simulink model "Cessna_6DOF_Wind_trim"  (Simulink 8.6)
settings: Solver=ode45  StartTime=0.0  StopTime=10.0  RelTol=1e-3
values from neighbouring files (symbols this model uses):
  alpha = alpha_delta_e_thrust(1,1)    [Initial_Cessna.m]
  beta = 0    [Initial_Cessna.m]
  I_xx = 1285.31    [Initial_Cessna.m]
  I_yy = 1824.93    [Initial_Cessna.m]
  I_zz = 2666.893    [Initial_Cessna.m]
  p = 0    [Initial_Cessna.m]
  q = 0    [Initial_Cessna.m]
  r = 0    [Initial_Cessna.m]
  V = 60    [Initial_Cessna.m]    (also in Trim_Cessna_Body.m)
  x = 0    [Initial_Cessna.m]
  y = 0    [Initial_Cessna.m]
  z = 0    [Initial_Cessna.m]
libraries: aerolibobsolete x1
settings Model: Creator=Pranav  LastModifiedBy=siddharth
settings DebuggingCC: FcnCallInpInsideContextMsg=UseLocalSettings
settings ConfigComp: CovSFcnEnable=off

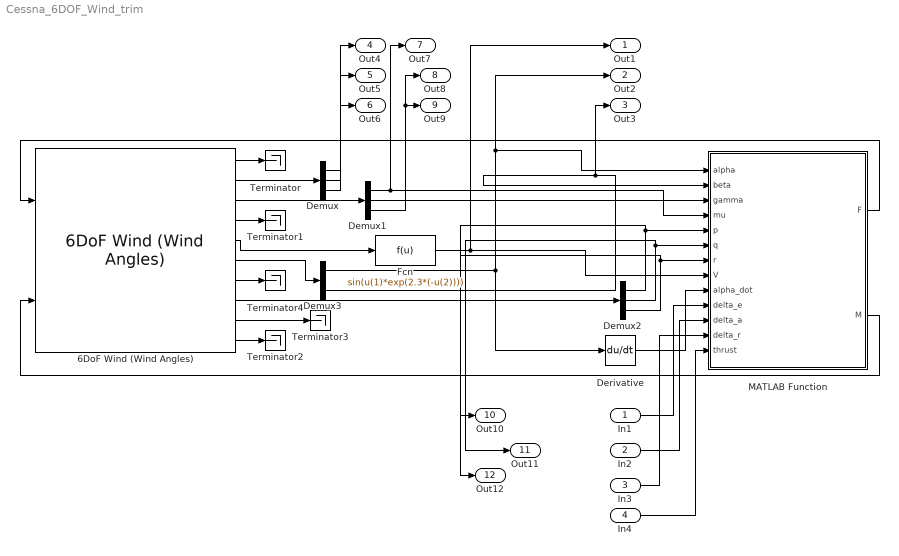
== system Cessna_6DOF_Wind_trim ==
  In1 : Inport
  In2 : Inport  Port=2
  In3 : Inport  Port=3
  In4 : Inport  Port=4
  6DoF Wind (Wind Angles) : aerolibobsolete/6DoF Wind (Wind Angles)  units=Metric (MKS)  mtype=Fixed  rep=Wind Angles  xme_0=[x y z]  Vm_0=[V alpha beta]  wind_0=[0 0 0]  pm_0=[p q r]  mass_0=m  mass_e=0.5  mass_f=2.0  inertia=diag([I_xx I_yy I_zz])  inertia_e=eye(3)  inertia_f=2*eye(3)
  Demux : Demux  Outputs=3
  Demux1 : Demux  Outputs=3
  Demux2 : Demux  Outputs=3
  Demux3 : Demux  Outputs=2
  Derivative : Derivative
  Fcn : Fcn  Expr=sin(u(1)*exp(2.3*(-u(2))))
  MATLAB Function : MATLAB Function  TreatAsAtomicUnit=on
  Terminator{,1..4} (5 alike) : Terminator
  Out1 : Outport
  Out2 : Outport  Port=2
  Out3 : Outport  Port=3
  Out4 : Outport  Port=4
  Out5 : Outport  Port=5
  Out6 : Outport  Port=6
  Out7 : Outport  Port=7
  Out8 : Outport  Port=8
  Out9 : Outport  Port=9
  Out10 : Outport  Port=10
  Out11 : Outport  Port=11
  Out12 : Outport  Port=12
  wires:
  MATLAB Function/1(F) -> 6DoF Wind (Wind Angles)/1
  MATLAB Function/2(M) -> 6DoF Wind (Wind Angles)/2
  6DoF Wind (Wind Angles)/2 -> Demux/1
  6DoF Wind (Wind Angles)/1 -> Terminator/1
  6DoF Wind (Wind Angles)/3 -> Demux1/1
  6DoF Wind (Wind Angles)/4 -> Terminator1/1
  6DoF Wind (Wind Angles)/10 -> Terminator2/1
  6DoF Wind (Wind Angles)/9 -> Terminator3/1
  6DoF Wind (Wind Angles)/8 -> Demux2/1
  6DoF Wind (Wind Angles)/7 -> Terminator4/1
  6DoF Wind (Wind Angles)/6 -> Demux3/1
  Demux3/1 -> Derivative/1, MATLAB Function/1(alpha), Out2/1
  Demux2/1 -> Out10/1, MATLAB Function/5(p)
  Demux2/2 -> Out11/1, MATLAB Function/6(q)
  Demux2/3 -> Out12/1, MATLAB Function/7(r)
  Demux3/2 -> MATLAB Function/2(beta), Out3/1
  Demux1/1 -> MATLAB Function/4(mu), Out7/1
  Demux1/2 -> MATLAB Function/3(gamma)
  6DoF Wind (Wind Angles)/5 -> Fcn/1
  Fcn/1 -> MATLAB Function/8(V), Out1/1
  Derivative/1 -> MATLAB Function/9(alpha_dot)
  In1/1 -> MATLAB Function/10(delta_e)
  In2/1 -> MATLAB Function/11(delta_a)
  In3/1 -> MATLAB Function/12(delta_r)
  In4/1 -> MATLAB Function/13(thrust)
  Demux/1 -> Out4/1
  Demux/2 -> Out5/1
  Demux/3 -> Out6/1
  Demux1/3 -> Out9/1, Out8/1

== matlab function MATLAB Function ==
  data: alpha input double; F output double; beta input double; gamma input double; mu input double; p input double; q input double; r input double; V input double; alpha_dot input double; M output double; delta_e input double; delta_a input double; delta_r input double; thrust input double
function [F, M] = Force_Cessna(alpha, beta, gamma, mu, p, q, r, V, alpha_dot, delta_e, delta_a, delta_r, thrust)

g = 9.8;
rho = 1.225;

m = 1043.26;
C_bar = 1.493;
b = 10.911;
S_ref = 16.1651;

C_L_0 = 0.25;
C_L_alpha = 4.47;
C_L_q = 1.7;
C_L_delta_e = 0.3476;

C_D_0 = 0.036;
C_D_alpha = 0.13;
C_D_beta = 0.17;
C_D_delta_e = 0.06;

C_Y_beta = -0.31;
C_Y_p = -0.037;
C_Y_r = 0.21;
C_Y_delta_a = 0;

C_l_beta = -0.089;
C_l_p = -0.47;
C_l_r = 0.096;
C_l_delta_a = -0.09;
C_l_delta_r = 0.0147;

C_M_0 = -0.02;
C_M_alpha = -1.8;
C_M_alpha_dot = -12.4;
C_M_delta_e = -1.28;

C_N_beta = 0.065;
C_N_p = -0.03;
C_N_r = -0.99;
C_N_delta_a = -0.0053;
C_N_delta_r = -0.0657;

% delta_e = -0.0304;
% delta_a = 0;
% delta_r = 0;
% thrust = 1397;

C_L = C_L_0 + C_L_alpha*alpha + C_L_q*(q*C_bar/(2*V)) + C_L_delta_e*delta_e;
C_D = C_D_0 + C_D_alpha*abs(alpha) + C_D_beta*abs(beta) + C_D_delta_e*abs(delta_e);
C_Y = C_Y_beta*beta + C_Y_p*(p*b/(2*V)) + C_Y_r*(r*b/(2*V)) + C_Y_delta_a*delta_a;

C_l = C_l_beta*beta + C_l_p*(p*b/(2*V)) + C_l_r*(r*b/(2*V)) + C_l_delta_a*delta_a + C_l_delta_r*delta_r;
C_M = C_M_0 + C_M_alpha*alpha + C_M_alpha_dot*(alpha_dot*C_bar/(2*V)) + C_M_delta_e*delta_e;
C_N = C_N_beta*beta + C_N_p*(p*b/(2*V)) + C_N_r*(r*b/(2*V)) + C_N_delta_a*delta_a + C_N_delta_r*delta_r;

F = zeros(3,1);
M = zeros(3,1);

q_bar = 0.5*rho*V*V;

F(1,1) = q_bar*S_ref*(-C_D*cos(beta) + C_Y*sin(beta)) - m*g*sin(gamma) + thrust*cos(alpha)*cos(beta);
F(2,1) = q_bar*S_ref*(C_D*sin(beta) + C_Y*sin(beta)) - m*g*cos(gamma)*sin(mu) - thrust*cos(alpha)*sin(beta);
F(3,1) = q_bar*S_ref*(-C_L) + m*g*cos(gamma)*cos(mu) - thrust*sin(alpha);

M(1,1) = q_bar*S_ref*b*C_l;
M(2,1) = q_bar*S_ref*C_bar*C_M;
M(3,1) = q_bar*S_ref*b*C_N;
